simulink model "Copter_Plane_V10_sim"  (R2021a)
settings: Solver=ode1  StartTime=0.0  StopTime=10  FixedStep=dt  RelTol=1e-3
undefined symbols (not defined in the file or in its folder): AC_Attitude, AC_PosControl, accel_target, AP_Motors, curr_pos, Curr_sate, curr_vel, Euler, GRAVITY_MSS, gyro, HD, J, m_kg, Newton, pid_vel_xy_input, pos_target, position, Raphson, rho, SINS, SRV_Channel, Vehicle, vel_target, velocity
libraries: sharedutil x4, shared6dofsys x2, simulink x2, sharedtransform x2, aerolibasang x1
(part 2 of 2)

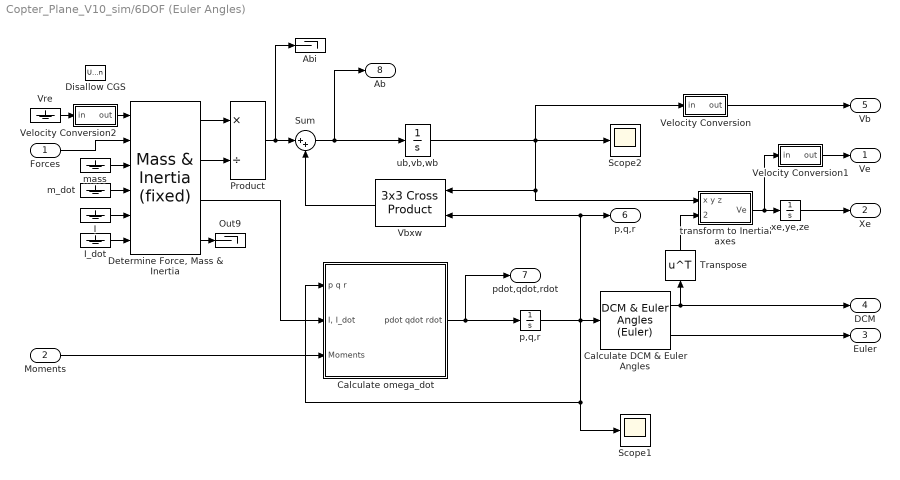
== system Copter_Plane_V10_sim/6DOF (Euler Angles) ==
  Forces : Inport  Unit=N  PortDimensions=3
  Moments : Inport  Port=2  Unit=N*m  PortDimensions=3
  Abi : Terminator
  Calculate DCM & Euler Angles : shared6dofsys/DCM & Euler Angles (Euler)  aMode=aMode
      settings: SourceProductBaseCode=AE,PW,DR,MT,UV,VE
  Calculate omega_dot : Subsystem  AncestorBlock=shared6dofsys/Calculate omega_dot  mask{aMode=aMode}
      mask init:
      | if aerosharedtest(gcb)
      |     aerosharedicon('shared');
      | else
      |     sharedautoicon('shared');
      | end
  "Determine Force, Mass & Inertia" : shared6dofsys/Mass & Inertia (fixed)  aMode=aMode
      settings: SourceProductBaseCode=AE,PW,DR,MT,UV,VE
  Disallow CGS : UnitConfiguration  UnitSystemsStr=English,SI,SI (extended)  AllowAllUnitSystems=off
  I : Ground
  I_dot : Ground
  Out9 : Terminator
  Product : Product  Inputs=*/  SaturateOnIntegerOverflow=on  OutDataTypeStr=Inherit: Same as first input
  Scope1 : Scope
  Scope2 : Scope
  Sum : Sum  Inputs=|++  SaturateOnIntegerOverflow=on
  Transpose : Math  Operator=transpose  SignedPower=on  SaturateOnIntegerOverflow=on
  Vbxw : sharedutil/3x3 Cross Product  aMode=aMode
      settings: SourceProductBaseCode=AE,PW,DR,MT,UV,VE
  Velocity Conversion : Subsystem
  Velocity Conversion1 : Subsystem
  Velocity Conversion2 : Subsystem
  Vre : Ground
  m_dot : Ground
  mass : Ground
  "p,q,r " : Integrator  InitialCondition=pm_0  ContinuousStateAttributes=pm_statename
  "transform to Inertial axes " : Subsystem  mask(Vector Transformation){}
      mask Display: disp('L_EB')
  ub,vb,wb : Integrator  InitialCondition=Vm_0  ContinuousStateAttributes=Vm_statename
  xe,ye,ze : Integrator  InitialCondition=xme_0  ContinuousStateAttributes=xme_statename
  Ve : Outport  Unit=m/s  VectorParamsAs1DForOutWhenUnconnected=off
  Xe : Outport  Port=2  Unit=m  VectorParamsAs1DForOutWhenUnconnected=off
  Euler : Outport  Port=3  Unit=rad  VectorParamsAs1DForOutWhenUnconnected=off
  DCM : Outport  Port=4  Unit=1  VectorParamsAs1DForOutWhenUnconnected=off
  Vb : Outport  Port=5  Unit=m/s  VectorParamsAs1DForOutWhenUnconnected=off
  p,q,r : Outport  Port=6  Unit=rad/s  VectorParamsAs1DForOutWhenUnconnected=off
  pdot,qdot,rdot : Outport  Port=7  Unit=rad/s^2  VectorParamsAs1DForOutWhenUnconnected=off
  Ab : Outport  Port=8  Unit=m/s^2  VectorParamsAs1DForOutWhenUnconnected=off
  wires:
  Velocity Conversion1/1(out) -> Ve/1
  Sum/1 -> Ab/1, ub,vb,wb/1
  ub,vb,wb/1 -> "transform to Inertial axes "/1(x y z), Vbxw/1, Scope2/1, Velocity Conversion/1(in)
  Velocity Conversion/1(out) -> Vb/1
  Velocity Conversion2/1(out) -> "Determine Force, Mass & Inertia"/1
  Vre/1 -> Velocity Conversion2/1(in)
  "Determine Force, Mass & Inertia"/1 -> Product/1
  I_dot/1 -> "Determine Force, Mass & Inertia"/6
  I/1 -> "Determine Force, Mass & Inertia"/5
  Calculate omega_dot/1(pdot qdot rdot) -> "p,q,r "/1, pdot,qdot,rdot/1
  "Determine Force, Mass & Inertia"/4 -> Out9/1
  m_dot/1 -> "Determine Force, Mass & Inertia"/4
  "Determine Force, Mass & Inertia"/2 -> Product/2
  mass/1 -> "Determine Force, Mass & Inertia"/3
  Transpose/1 -> "transform to Inertial axes "/2(transform coefficients)
  Calculate DCM & Euler Angles/1 -> Transpose/1, DCM/1
  Product/1 -> Sum/1, Abi/1
  Forces/1 -> "Determine Force, Mass & Inertia"/2
  Moments/1 -> Calculate omega_dot/3(Moments)
  "p,q,r "/1 -> Calculate DCM & Euler Angles/1, Scope1/1, Calculate omega_dot/1(p q r), p,q,r/1, Vbxw/2
  "transform to Inertial axes "/1(Ve) -> xe,ye,ze/1, Velocity Conversion1/1(in)
  xe,ye,ze/1 -> Xe/1
  Vbxw/1 -> Sum/2
  Calculate DCM & Euler Angles/2 -> Euler/1
  "Determine Force, Mass & Inertia"/3 -> Calculate omega_dot/2("I, I_dot")

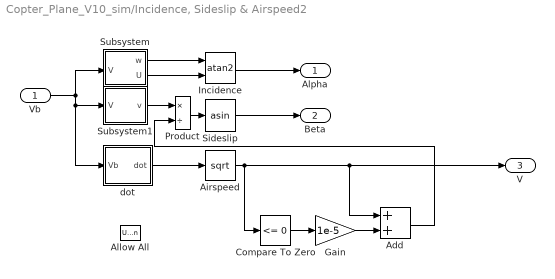
== system Copter_Plane_V10_sim/Incidence, Sideslip & Airspeed2 ==
  Vb : Inport
  Add : Sum
  Airspeed : Sqrt  AlgorithmType=Newton-Raphson  SaturateOnIntegerOverflow=on
  Allow All : UnitConfiguration  UnitSystemsStr=English,SI,SI (extended)  AllowAllUnitSystems=off
  Compare To Zero : simulink/Logic and Bit Operations/Compare To Zero  relop=<=  OutDataTypeStr=boolean
  Gain : Gain  Gain=1e-5
  Incidence : Trigonometry  Operator=atan2
  Product : Product  Inputs=*/  SaturateOnIntegerOverflow=on  OutDataTypeStr=Inherit: Same as first input
  Sideslip : Trigonometry  Operator=asin
  Subsystem : Subsystem
  Subsystem1 : Subsystem
  dot : Subsystem
  Alpha : Outport  Unit=rad  InitialOutput=0  VectorParamsAs1DForOutWhenUnconnected=off
  Beta : Outport  Port=2  Unit=rad  InitialOutput=0  VectorParamsAs1DForOutWhenUnconnected=off
  V : Outport  Port=3  InitialOutput=0  VectorParamsAs1DForOutWhenUnconnected=off
  wires:
  Product/1 -> Sideslip/1
  Subsystem/1(w) -> Incidence/1
  Subsystem/2(U) -> Incidence/2
  dot/1(dot) -> Airspeed/1
  Airspeed/1 -> Compare To Zero/1, Add/1, V/1
  Incidence/1 -> Alpha/1
  Vb/1 -> Subsystem/1(V), Subsystem1/1(V), dot/1(Vb)
  Sideslip/1 -> Beta/1
  Subsystem1/1(v) -> Product/1
  Compare To Zero/1 -> Gain/1
  Gain/1 -> Add/2
  Add/1 -> Product/2

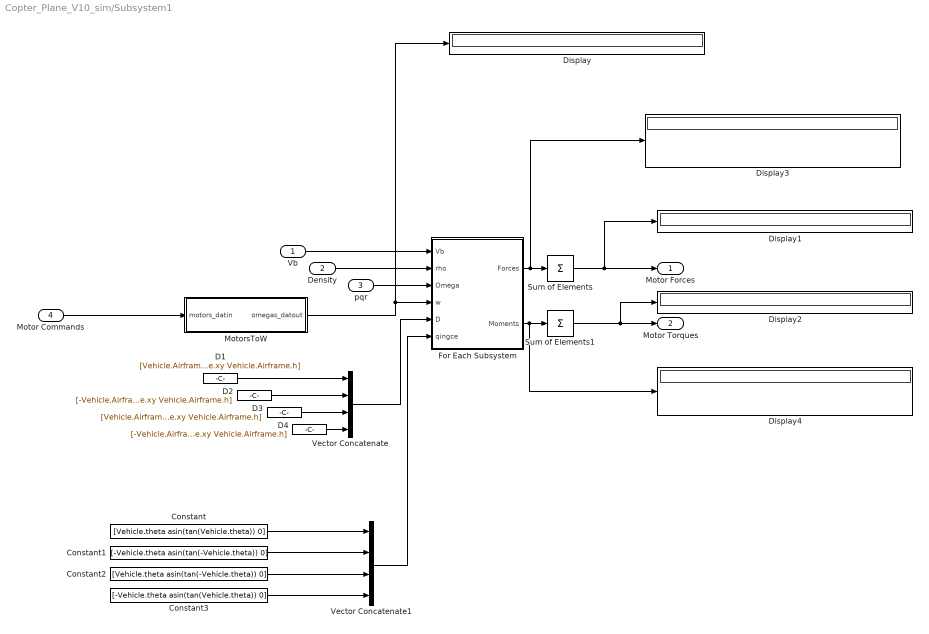
== system Copter_Plane_V10_sim/Subsystem1 ==
  Vb : Inport
  Density : Inport  Port=2
  pqr : Inport  Port=3
  Motor Commands : Inport  Port=4
  Constant : Constant  Value=[Vehicle.theta asin(tan(Vehicle.theta)) 0]
  Constant1 : Constant  Value=[-Vehicle.theta asin(tan(-Vehicle.theta)) 0]
  Constant2 : Constant  Value=[Vehicle.theta asin(tan(-Vehicle.theta)) 0]
  Constant3 : Constant  Value=[-Vehicle.theta asin(tan(Vehicle.theta)) 0]
  D1 : Constant  Value=[Vehicle.Airframe.xy +Vehicle.Airframe.xy Vehicle.Airframe.h]
  D2 : Constant  Value=[-Vehicle.Airframe.xy -Vehicle.Airframe.xy Vehicle.Airframe.h]
  D3 : Constant  Value=[Vehicle.Airframe.xy -Vehicle.Airframe.xy Vehicle.Airframe.h]
  D4 : Constant  Value=[-Vehicle.Airframe.xy Vehicle.Airframe.xy Vehicle.Airframe.h]
  Display{,1..4} (5 alike) : Display
  For Each Subsystem : Subsystem  TreatAsAtomicUnit=on
  MotorsToW : Subsystem
  Sum of Elements : Sum  Inputs=+  CollapseMode=Specified dimension  CollapseDim=2
  Sum of Elements1 : Sum  Inputs=+  CollapseMode=Specified dimension  CollapseDim=2
  Vector Concatenate : Concatenate  NumInputs=4  Mode=Multidimensional array  ConcatenateDimension=2
  Vector Concatenate1 : Concatenate  NumInputs=4  Mode=Multidimensional array  ConcatenateDimension=2
  Motor Forces : Outport  Unit=N  VectorParamsAs1DForOutWhenUnconnected=off
  Motor Torques : Outport  Port=2  Unit=N*m  VectorParamsAs1DForOutWhenUnconnected=off
  wires:
  Vector Concatenate/1 -> For Each Subsystem/5(D)
  Density/1 -> For Each Subsystem/2(rho)
  D4/1 -> Vector Concatenate/4
  Vb/1 -> For Each Subsystem/1(Vb)
  Sum of Elements1/1 -> Display2/1, Motor Torques/1
  D3/1 -> Vector Concatenate/3
  Sum of Elements/1 -> Display1/1, Motor Forces/1
  pqr/1 -> For Each Subsystem/3(Omega)
  D1/1 -> Vector Concatenate/1
  For Each Subsystem/2(Moments) -> Display4/1, Sum of Elements1/1
  For Each Subsystem/1(Forces) -> Display3/1, Sum of Elements/1
  D2/1 -> Vector Concatenate/2
  MotorsToW/1(omegas_datout) -> Display/1, For Each Subsystem/4(w)
  Motor Commands/1 -> MotorsToW/1(motors_datin)
  Vector Concatenate1/1 -> For Each Subsystem/6(qingce)
  Constant/1 -> Vector Concatenate1/1
  Constant1/1 -> Vector Concatenate1/2
  Constant2/1 -> Vector Concatenate1/3
  Constant3/1 -> Vector Concatenate1/4

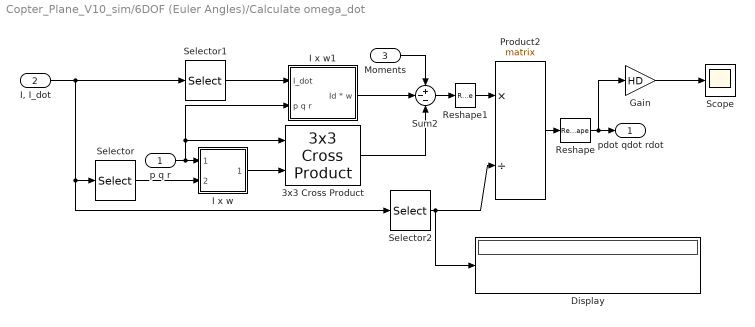
== system Copter_Plane_V10_sim/6DOF (Euler Angles)/Calculate omega_dot ==
  p q r : Inport
  "I, I_dot" : Inport  Port=2
  Moments : Inport  Port=3
  3x3 Cross Product : sharedutil/3x3 Cross Product  aMode=aMode
      settings: SourceProductBaseCode=AE,PW,DR,MT,UV,VE
  Display : Display
  Gain : Gain  Gain=HD
  I x w : Subsystem
  I x w1 : Subsystem
  Product2 : Product  Inputs=*/  Multiplication=Matrix(*)  SaturateOnIntegerOverflow=on  OutDataTypeStr=Inherit: Same as first input
  Reshape : Reshape
  Reshape1 : Reshape  OutputDimensionality=Row vector (2-D)
  Scope : Scope
  Selector : Selector  NumberOfDimensions=2  InputPortWidth=2  IndexOptions=Index vector (dialog),Select all  Indices=1:3,-1  OutputSizes=1
  Selector1 : Selector  NumberOfDimensions=2  InputPortWidth=2  IndexOptions=Index vector (dialog),Select all  Indices=4:6,-1  OutputSizes=1
  Selector2 : Selector  NumberOfDimensions=2  InputPortWidth=2  IndexOptions=Index vector (dialog),Select all  Indices=1:3,-1  OutputSizes=1
  Sum2 : Sum  Inputs=+--  SaturateOnIntegerOverflow=on
  pdot qdot rdot : Outport  VectorParamsAs1DForOutWhenUnconnected=off
  wires:
  Reshape1/1 -> Product2/1
  I x w/1(I * w) -> 3x3 Cross Product/2
  3x3 Cross Product/1 -> Sum2/3
  Selector1/1 -> I x w1/1(I_dot)
  I x w1/1(Id * w) -> Sum2/2
  Moments/1 -> Sum2/1
  Sum2/1 -> Reshape1/1
  Product2/1 -> Reshape/1
  p q r/1 -> I x w1/2(p q r), 3x3 Cross Product/1, I x w/1(p q r)
  "I, I_dot"/1 -> Selector1/1, Selector2/1, Selector/1
  Selector/1 -> I x w/2(Inertia)
  Reshape/1 -> Gain/1, pdot qdot rdot/1
  Selector2/1 -> Display/1, Product2/2
  Gain/1 -> Scope/1

== system Copter_Plane_V10_sim/6DOF (Euler Angles)/Velocity Conversion ==
  in : Inport  Unit=m/s
  Unit Conversion : UnitConversion
  out : Outport  VectorParamsAs1DForOutWhenUnconnected=off
  wires:
  Unit Conversion/1 -> out/1
  in/1 -> Unit Conversion/1

== system Copter_Plane_V10_sim/6DOF (Euler Angles)/Velocity Conversion1 ==
  in : Inport  Unit=m/s
  Unit Conversion : UnitConversion
  out : Outport  VectorParamsAs1DForOutWhenUnconnected=off
  wires:
  Unit Conversion/1 -> out/1
  in/1 -> Unit Conversion/1

== system Copter_Plane_V10_sim/6DOF (Euler Angles)/Velocity Conversion2 ==
  in : Inport  Unit=m/s
  Unit Conversion : UnitConversion
  out : Outport  Unit=m/s  VectorParamsAs1DForOutWhenUnconnected=off
  wires:
  Unit Conversion/1 -> out/1
  in/1 -> Unit Conversion/1

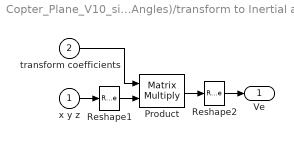
== system Copter_Plane_V10_sim/6DOF (Euler Angles)/transform to Inertial axes  ==
  x y z : Inport
  transform coefficients : Inport  Port=2
  Product : Product  Multiplication=Matrix(*)  InputSameDT=on  SaturateOnIntegerOverflow=on  OutDataTypeStr=Inherit: Same as first input
  Reshape1 : Reshape  OutputDimensionality=Column vector (2-D)
  Reshape2 : Reshape
  Ve : Outport  VectorParamsAs1DForOutWhenUnconnected=off
  wires:
  Reshape2/1 -> Ve/1
  Reshape1/1 -> Product/2
  x y z/1 -> Reshape1/1
  transform coefficients/1 -> Product/1
  Product/1 -> Reshape2/1

== system Copter_Plane_V10_sim/Incidence, Sideslip & Airspeed2/Subsystem ==
  V : Inport
  Demux1 : Demux  Outputs=3
      settings: DisplayOption=none
  Terminator : Terminator
  w : Outport  VectorParamsAs1DForOutWhenUnconnected=off
  U : Outport  Port=2  VectorParamsAs1DForOutWhenUnconnected=off
  wires:
  Demux1/3 -> w/1
  Demux1/2 -> Terminator/1
  V/1 -> Demux1/1
  Demux1/1 -> U/1

== system Copter_Plane_V10_sim/Incidence, Sideslip & Airspeed2/Subsystem1 ==
  V : Inport
  Demux1 : Demux  Outputs=3
      settings: DisplayOption=none
  Terminator : Terminator
  Terminator1 : Terminator
  v : Outport  VectorParamsAs1DForOutWhenUnconnected=off
  wires:
  Demux1/1 -> Terminator/1
  Demux1/3 -> Terminator1/1
  V/1 -> Demux1/1
  Demux1/2 -> v/1

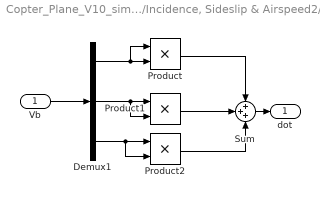
== system Copter_Plane_V10_sim/Incidence, Sideslip & Airspeed2/dot ==
  Vb : Inport
  Demux1 : Demux  Outputs=3
  Product : Product  RndMeth=Zero
  Product1 : Product  RndMeth=Zero
  Product2 : Product  RndMeth=Zero
  Sum : Sum  Inputs=+++
  dot : Outport  VectorParamsAs1DForOutWhenUnconnected=off
  wires:
  Product2/1 -> Sum/3
  Demux1/3 -> Product2/2, Product2/1
  Product/1 -> Sum/1
  Product1/1 -> Sum/2
  Sum/1 -> dot/1
  Vb/1 -> Demux1/1
  Demux1/1 -> Product/2, Product/1
  Demux1/2 -> Product1/1, Product1/2

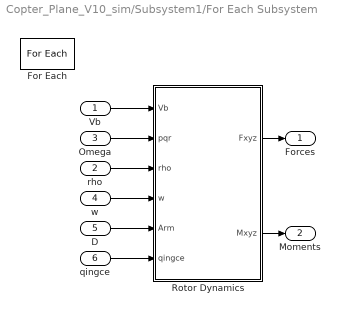
== system Copter_Plane_V10_sim/Subsystem1/For Each Subsystem ==
  Vb : Inport  PortDimensions=3
  rho : Inport  Port=2  PortDimensions=1
  Omega : Inport  Port=3
  w : Inport  Port=4  Partition=on  PartitionDimension=2  PartitionWidth=1  PartitionOffset=0
  D : Inport  Port=5  Partition=on  PartitionDimension=2  PartitionWidth=1  PartitionOffset=0
  qingce : Inport  Port=6  Partition=on  PartitionDimension=2  PartitionWidth=1  PartitionOffset=0
  For Each : ForEach  DisableCoverage=on
  Rotor Dynamics : Subsystem  AncestorBlock=dynamicsLibrary/Rotor Dynamics  TreatAsAtomicUnit=on
      mask init:
      | aeroicon('aeroblk');
      settings: RTWFcnNameOpts=Use subsystem name  RTWFileNameOpts=Use function name
  Forces : Outport  ConcatenationDimension=2  VectorParamsAs1DForOutWhenUnconnected=off
  Moments : Outport  Port=2  ConcatenationDimension=2  VectorParamsAs1DForOutWhenUnconnected=off
  wires:
  Rotor Dynamics/1(Fxyz) -> Forces/1
  Rotor Dynamics/2(Mxyz) -> Moments/1
  Vb/1 -> Rotor Dynamics/1(Vb)
  Omega/1 -> Rotor Dynamics/2(pqr)
  rho/1 -> Rotor Dynamics/3(rho)
  D/1 -> Rotor Dynamics/5(Arm)
  w/1 -> Rotor Dynamics/4(w)
  qingce/1 -> Rotor Dynamics/6(qingce)

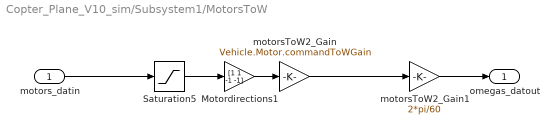
== system Copter_Plane_V10_sim/Subsystem1/MotorsToW ==
  motors_datin : Inport
  Motordirections1 : Gain  Gain=[1 1 -1 -1]  ParamDataTypeStr=single  OutDataTypeStr=Inherit: Inherit via back propagation  SaturateOnIntegerOverflow=on
  Saturation5 : Saturate  UpperLimit=1  LowerLimit=realmin  OutDataTypeStr=Inherit: Inherit via back propagation
  motorsToW2_Gain : Gain  Gain=Vehicle.Motor.commandToWGain  ParamDataTypeStr=single  OutDataTypeStr=Inherit: Inherit via back propagation  SaturateOnIntegerOverflow=on
  motorsToW2_Gain1 : Gain  Gain=2*pi/60  ParamDataTypeStr=single  OutDataTypeStr=Inherit: Inherit via back propagation  SaturateOnIntegerOverflow=on
  omegas_datout : Outport  VectorParamsAs1DForOutWhenUnconnected=off
  wires:
  Saturation5/1 -> Motordirections1/1
  Motordirections1/1 -> motorsToW2_Gain/1
  motors_datin/1 -> Saturation5/1
  motorsToW2_Gain/1 -> motorsToW2_Gain1/1
  motorsToW2_Gain1/1 -> omegas_datout/1

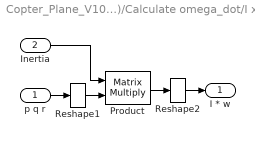
== system Copter_Plane_V10_sim/6DOF (Euler Angles)/Calculate omega_dot/I x w ==
  p q r : Inport
  Inertia : Inport  Port=2
  Product : Product  Multiplication=Matrix(*)  InputSameDT=on  SaturateOnIntegerOverflow=on  OutDataTypeStr=Inherit: Same as first input
  Reshape1 : Reshape  OutputDimensionality=Column vector (2-D)
  Reshape2 : Reshape
  I * w : Outport  VectorParamsAs1DForOutWhenUnconnected=off
  wires:
  Reshape2/1 -> I * w/1
  Reshape1/1 -> Product/2
  p q r/1 -> Reshape1/1
  Inertia/1 -> Product/1
  Product/1 -> Reshape2/1

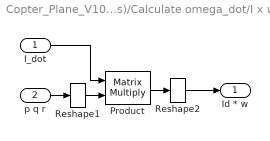
== system Copter_Plane_V10_sim/6DOF (Euler Angles)/Calculate omega_dot/I x w1 ==
  I_dot : Inport
  p q r : Inport  Port=2
  Product : Product  Multiplication=Matrix(*)  InputSameDT=on  SaturateOnIntegerOverflow=on  OutDataTypeStr=Inherit: Same as first input
  Reshape1 : Reshape  OutputDimensionality=Column vector (2-D)
  Reshape2 : Reshape
  Id * w : Outport  VectorParamsAs1DForOutWhenUnconnected=off
  wires:
  Reshape2/1 -> Id * w/1
  Reshape1/1 -> Product/2
  Product/1 -> Reshape2/1
  I_dot/1 -> Product/1
  p q r/1 -> Reshape1/1

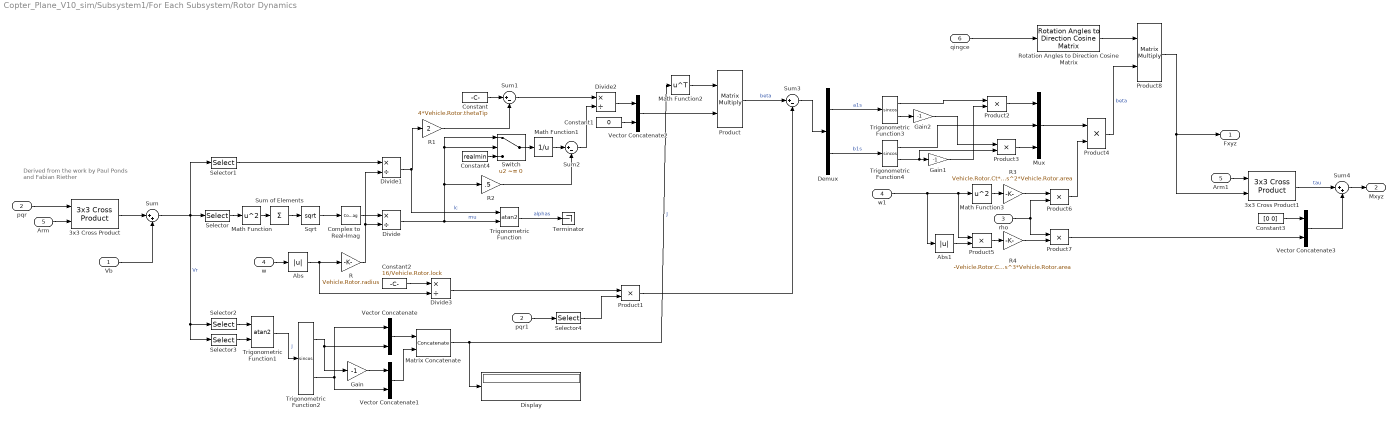
== system Copter_Plane_V10_sim/Subsystem1/For Each Subsystem/Rotor Dynamics ==
  note: Derived from the work by Paul Ponds
      | and Fabian Riether
  Vb : Inport  PortDimensions=3
  pqr : Inport  Port=2  PortDimensions=3
  rho : Inport  Port=3  PortDimensions=1
  w : Inport  Port=4  PortDimensions=[1 1]
  Arm : Inport  Port=5  PortDimensions=[3 1]
  qingce : Inport  Port=6  PortDimensions=[3 1]
  3x3 Cross Product : sharedutil/3x3 Cross Product  aMode=aMode
      settings: SourceProductBaseCode=AE,PW,DR,MT,UV,VE
  3x3 Cross Product1 : sharedutil/3x3 Cross Product  aMode=aMode
      settings: SourceProductBaseCode=AE,PW,DR,MT,UV,VE
  Abs : Abs
  Abs1 : Abs
  Arm1 : InportShadow  Port=5  PortDimensions=[3 1]
  Complex to Real-Imag : ComplexToRealImag  Output=Real
  Constant : Constant  Value=4*Vehicle.Rotor.thetaTip
  Constant1 : Constant  Value=0
  Constant2 : Constant  Value=16/Vehicle.Rotor.lock
  Constant3 : Constant  Value=[0 0]
  Constant4 : Constant  Value=realmin
  Demux : Demux  Outputs=2
  Display : Display
  Divide{,1..3} (4 alike) : Product  Inputs=*/
  Gain : Gain  Gain=-1
  Gain1 : Gain  Gain=-1
  Gain2 : Gain  Gain=-1
  Math Function : Math  Operator=square  SignedPower=on  SaturateOnIntegerOverflow=on
  Math Function1 : Math  Operator=reciprocal  SignedPower=on  SaturateOnIntegerOverflow=on
  Math Function2 : Math  Operator=transpose  SignedPower=on  SaturateOnIntegerOverflow=on
  Math Function3 : Math  Operator=square  SignedPower=on  SaturateOnIntegerOverflow=on
  Matrix Concatenate : Concatenate  Mode=Multidimensional array  ConcatenateDimension=2
  Mux : Mux  Inputs=3
  Product : Product  Multiplication=Matrix(*)
  Product{1..7} (7 alike) : Product
  Product8 : Product  Multiplication=Matrix(*)
  R : Gain  Gain=Vehicle.Rotor.radius
  R1 : Gain  Gain=2
  R2 : Gain  Gain=.5
  R3 : Gain  Gain=Vehicle.Rotor.Ct*Vehicle.Rotor.radius^2*Vehicle.Rotor.area
  R4 : Gain  Gain=-Vehicle.Rotor.Cq*Vehicle.Rotor.radius^3*Vehicle.Rotor.area
  Rotation Angles to Direction Cosine Matrix : sharedtransform/Rotation Angles to Direction Cosine Matrix  rotationOrder=YXZ  aMode=aMode
      settings: SourceProductBaseCode=AE,PW,DR,MT,UV,VE
  Selector : Selector  InputPortWidth=3  IndexOptions=Index vector (dialog)  Indices=[1 2]  OutputSizes=1
  Selector1 : Selector  InputPortWidth=3  IndexOptions=Index vector (dialog)  Indices=[3]  OutputSizes=1
  Selector2 : Selector  InputPortWidth=3  IndexOptions=Index vector (dialog)  Indices=[2]  OutputSizes=1
  Selector3 : Selector  InputPortWidth=3  IndexOptions=Index vector (dialog)  Indices=[1]  OutputSizes=1
  Selector4 : Selector  InputPortWidth=3  IndexOptions=Index vector (dialog)  Indices=[2 1]  OutputSizes=1
  Sqrt : Sqrt  OutputSignalType=complex  SaturateOnIntegerOverflow=on
  Sum : Sum  Inputs=|++
  Sum of Elements : Sum  Inputs=+
  Sum1 : Sum  Inputs=|+-
  Sum2 : Sum  Inputs=|+-
  Sum3 : Sum  Inputs=|+-
  Sum4 : Sum  Inputs=|++
  Switch : Switch  Criteria=u2 ~= 0
  Terminator : Terminator
  Trigonometric Function : Trigonometry  Operator=atan2
  Trigonometric Function1 : Trigonometry  Operator=atan2
  Trigonometric Function2 : Trigonometry  Operator=sincos
  Trigonometric Function3 : Trigonometry  Operator=sincos
  Trigonometric Function4 : Trigonometry  Operator=sincos
  Vector Concatenate{,1..3} (4 alike) : Concatenate
  pqr1 : InportShadow  Port=2  PortDimensions=3
  w1 : InportShadow  Port=4  PortDimensions=[1 1]
  Fxyz : Outport  PortDimensions=[3 1]  VectorParamsAs1DForOutWhenUnconnected=off
  Mxyz : Outport  Port=2  PortDimensions=[3 1]  VectorParamsAs1DForOutWhenUnconnected=off
  wires:
  Complex to Real-Imag/1 -> Divide/1
  Sqrt/1 -> Complex to Real-Imag/1
  Constant4/1 -> Switch/3
  Switch/1 -> Math Function1/1
  Product1/1 -> Sum3/2
  rho/1 -> Product7/1, Product6/2
  Product7/1 -> Vector Concatenate3/2
  Product6/1 -> Product4/2
  Sum4/1 -> Mxyz/1
  3x3 Cross Product1/1 -> Sum4/1  "tau"
  Arm1/1 -> 3x3 Cross Product1/1
  Vector Concatenate3/1 -> Sum4/2
  Constant3/1 -> Vector Concatenate3/1
  R4/1 -> Product7/2
  Product5/1 -> R4/1
  Abs1/1 -> Product5/2
  R3/1 -> Product6/1
  Mux/1 -> Product4/1
  Gain2/1 -> Product3/1
  Product3/1 -> Mux/3
  Trigonometric Function3/2 -> Gain2/1
  Trigonometric Function4/1 -> Mux/2
  Product2/1 -> Mux/1
  Trigonometric Function3/1 -> Product2/1
  Gain1/1 -> Product2/2
  Trigonometric Function4/2 -> Gain1/1, Product3/2
  Demux/2 -> Trigonometric Function4/1  "b1s"
  Demux/1 -> Trigonometric Function3/1  "a1s"
  Sum3/1 -> Demux/1
  Math Function3/1 -> R3/1
  w1/1 -> Math Function3/1, Product5/1, Abs1/1
  Divide3/1 -> Product1/1
  Abs/1 -> R/1, Divide3/2
  Selector4/1 -> Product1/2
  pqr1/1 -> Selector4/1
  Constant2/1 -> Divide3/1
  Product/1 -> Sum3/1  "beta"
  Math Function2/1 -> Product/1
  Vector Concatenate2/1 -> Product/2
  Constant1/1 -> Vector Concatenate2/2
  Divide2/1 -> Vector Concatenate2/1
  Sum2/1 -> Divide2/2
  R2/1 -> Sum2/2
  Math Function1/1 -> Sum2/1
  Sum1/1 -> Divide2/1
  R1/1 -> Sum1/2
  Constant/1 -> Sum1/1
  Matrix Concatenate/1 -> Display/1, Math Function2/1  "J"
  Vector Concatenate1/1 -> Matrix Concatenate/2
  Vector Concatenate/1 -> Matrix Concatenate/1
  Trigonometric Function2/1 -> Gain/1, Vector Concatenate/2
  Gain/1 -> Vector Concatenate1/1
  Trigonometric Function2/2 -> Vector Concatenate/1, Vector Concatenate1/2
  Trigonometric Function1/1 -> Trigonometric Function2/1  "j"
  Selector3/1 -> Trigonometric Function1/2
  Selector2/1 -> Trigonometric Function1/1
  Trigonometric Function/1 -> Terminator/1  "alphas"
  Divide1/1 -> Trigonometric Function/1, R1/1  "lc"
  Selector1/1 -> Divide1/1
  Divide/1 -> Trigonometric Function/2, Switch/1, Switch/2, R2/1  "mu"
  R/1 -> Divide/2, Divide1/2
  w/1 -> Abs/1
  Arm/1 -> 3x3 Cross Product/2
  pqr/1 -> 3x3 Cross Product/1
  Sum of Elements/1 -> Sqrt/1
  Math Function/1 -> Sum of Elements/1
  Selector/1 -> Math Function/1
  Sum/1 -> Selector/1, Selector1/1, Selector2/1, Selector3/1  "Vr"
  Vb/1 -> Sum/2
  3x3 Cross Product/1 -> Sum/1
  qingce/1 -> Rotation Angles to Direction Cosine Matrix/1
  Rotation Angles to Direction Cosine Matrix/1 -> Product8/1
  Product4/1 -> Product8/2  "beta"
  Product8/1 -> 3x3 Cross Product1/2, Fxyz/1

== matlab function Copter_Plane_V10_sim/MATLAB Function9 ==
  data: x_cmss input; forward output; y_cmss input; right output; yaw data_store_memory
function [forward, right]= to_body(  x_cmss,   y_cmss)  
global yaw
    forward = x_cmss * cos(yaw) + y_cmss * sin(yaw);
    right = -x_cmss * sin(yaw) + y_cmss * cos(yaw);

== matlab function Copter_Plane_V10_sim/MATLAB Function15 ==
  data: u input; y output
function y = fun(u)


y= to_euler(u);

== matlab function Copter_Plane_V10_sim/MATLAB Function16 ==
  data: u input; y output
function y = fun(u)

attitude_vehicle_quat=from_rotation_matrix(u);
y= to_euler(attitude_vehicle_quat);

== matlab function Copter_Plane_V10_sim/input_euler_angle_roll_pitch_euler_rate_yaw ==
  data: GRAVITY_MSS data_store_memory; HD data_store_memory; dt data_store_memory; LOCATION_SCALING_FACTOR_INV data_store_memory; PathModeOut_sl data_store_memory; plane_mode data_store_memory; algo_remote_ct_st data_store_memory; algo_dbg_param data_store_memory; Curr_sate data_store_memory; systime data_store_memory; Test_w data_store_memory; AC_rate_pitch_pid data_store_memory; AC_rate_roll_pid data_store_memory; AC_rate_yaw_pid data_store_memory; AC_PosControl data_store_memory; AP_rate_roll data_store_memory; AP_rate_pitch data_store_memory; AP_rate_yaw data_store_memory; AP_TECS data_store_memory; AP_L1 data_store_memory; Plane data_store_memory; SRV_Channel data_store_memory; AC_Attitude data_store_memory; AP_Motors data_store_memory; Copter_Plane data_store_memory; LOCATION_SCALING_FACTOR data_store_memory; SINS data_store_memory; SlewLimiter data_store_memory
function copter_plane_run
global plane_mode

run_remote();
load_Curr_sate();
loc_run();
load_inint();
sin_step_test();
    switch plane_mode
        case ENUM_plane_mode.V1000
            run_V1000();
        case {ENUM_plane_mode.V10 ,ENUM_plane_mode.V10s ,ENUM_plane_mode.V10_1}
            run_V10();
        otherwise
            run_V10();
    end 
run_servo_pwm_adj();

end

== matlab function Copter_Plane_V10_sim/MATLAB Function17 ==
  data: x_cmss input; forward output; y_cmss input; right output; SINS data_store_memory
function [forward, right]= to_body(  x_cmss,   y_cmss)  
global SINS
yaw =SINS.yaw;
    forward = x_cmss * cos(yaw) + y_cmss * sin(yaw);
    right = -x_cmss * sin(yaw) + y_cmss * cos(yaw);

== matlab function Copter_Plane_V10_sim/MATLAB Function ==
  data: PWM input; PWM_n output
function PWM_n      = fcn(PWM)

PWM_n=(PWM-1000)/1000;

== matlab function Copter_Plane_V10_sim/MATLAB Function1 ==
  data: k_rudder input; k_aileron input; k_throttle input; k_elevator input; wx input; wy input; wz input; alpha input; beta input; V input; Aero parameter; rho input; F output; M output
function [F,M] = fcn(k_rudder,k_aileron,k_throttle,k_elevator,wx,wy,wz,alpha,beta,V, Aero,rho)
% 
k_rudder=k_rudder/4500*30;
k_aileron=k_aileron/4500*30;
k_elevator=k_elevator/4500*30;
if(V<3)
    V=0;
end
V=0;
HD=180/pi;
% [~,~,rho,~] = atom_mode(alt+2000);
q=0.5*rho*V*V;
% alpha=constrain_value(alpha,-10/HD,12/HD);
% beta=constrain_value(beta,-10/HD,12/HD);
Sbw=[cos(alpha)*cos(beta)   -cos(alpha)*sin(beta)   -sin(alpha)
    sin(beta)               cos(beta)               0
    sin(alpha)*cos(beta)    -sin(alpha)*sin(beta)   cos(alpha)];
alpha=alpha*HD;
beta =beta* HD;
CL=interp1(Aero.CL_alpha,Aero.CL,alpha,'linear',0);
CD=interp1(Aero.CD_alpha,Aero.CD,alpha,'linear',0.25);
CC_beta=interp1(Aero.CC_beta,Aero.CC,abs(beta),'linear','extrap')*sign(beta);
CC=CC_beta+Aero.CC_dr*k_rudder;
D=q*Aero.Sref*CD;
C=q*Aero.Sref*CC;
L=q*Aero.Sref*CL;
Fw=[D; C; L];
Fb=Sbw*-Fw;
Fb=-Fw;
TF=k_throttle*Aero.Tmax;
F_Plane=Fb+[TF;0;0];

%%%%%%%%%%%%%%%%%%%%%%%%%%%%%%%%%%%%%%%%%%%%%%%%%%%%%%%%
% V-立尾
% H-平尾
% F-机身
% L-机翼

Cm_V=interp1(Aero.Cm_alpha,Aero.Cm_V,alpha,'linear','extrap');
Cm_H=interp1(Aero.Cm_alpha,Aero.Cm_H,alpha,'linear','extrap');
Cm_L=interp1(Aero.Cm_alpha,Aero.Cm_L,alpha,'linear','extrap');
Cm_F=interp1(Aero.Cm_alpha,Aero.Cm_F,alpha,'linear','extrap');
Cm_H_de=interp1(Aero.Cm_elevator,Aero.Cm_H_de,k_elevator,'linear','extrap');
Cm=Cm_V+Cm_H+Cm_L+Cm_F+Cm_H_de;

Cl_beta=interp1(Aero.beta,Aero.Cl_beta,abs(beta),'linear','extrap')*sign(beta);
Cl_da=Aero.Cl_da*k_aileron;
Cl=Cl_beta+Cl_da;

Cn_beta=interp1(Aero.beta,Aero.Cn_beta,abs(beta),'linear','extrap')*sign(beta);
Cn_dr=Aero.Cn_dr*k_rudder;
Cn=Cn_beta+Cn_dr;

l=q*Aero.Sref*Aero.Lref*Cl-0.1*wx;
m=q*Aero.Sref*Aero.Lref*Cm-0.3*wy;
n=q*Aero.Sref*Aero.Lref*Cn-0.2*wz;
M_Plane=[l ;m ;n];

F=F_Plane;
M=M_Plane;


end

== matlab function Copter_Plane_V10_sim/Location_offset1 ==
  data: center_WP input; current_loc output; ofs_north input; ofs_east input; LOCATION_SCALING_FACTOR_INV data_store_memory; HD data_store_memory
function current_loc=Location_offset( center_WP,ofs_north,  ofs_east)

current_loc=Location_offset( center_WP,ofs_north,  ofs_east);

== matlab function Copter_Plane_V10_sim/MATLAB Function2 ==
  data: x_cmss input; forward output; y_cmss input; right output; yaw data_store_memory
function [forward, right]= to_body(  x_cmss,   y_cmss)  
global yaw
    forward = x_cmss * cos(yaw) + y_cmss * sin(yaw);
    right = -x_cmss * sin(yaw) + y_cmss * cos(yaw);

== matlab function Copter_Plane_V10_sim/MATLAB Function3 ==
  data: x_cmss input; forward output; y_cmss input; right output; yaw data_store_memory
function [forward, right]= to_body(  x_cmss,   y_cmss)  
global yaw
    forward = x_cmss * cos(yaw) + y_cmss * sin(yaw);
    right = -x_cmss * sin(yaw) + y_cmss * cos(yaw);

== matlab function Copter_Plane_V10_sim/MATLAB Function4 ==
  data: x_cmss input; forward output; y_cmss input; right output; yaw data_store_memory
function [forward, right]= to_body(  x_cmss,   y_cmss)  
global yaw
    forward = x_cmss * cos(yaw) + y_cmss * sin(yaw);
    right = -x_cmss * sin(yaw) + y_cmss * cos(yaw);

== matlab function Copter_Plane_V10_sim/MATLAB Function6 ==
  data: x_cmss input; forward output; y_cmss input; right output; yaw data_store_memory
function [forward, right]= to_body(  x_cmss,   y_cmss)  
global yaw
    forward = x_cmss * cos(yaw) + y_cmss * sin(yaw);
    right = -x_cmss * sin(yaw) + y_cmss * cos(yaw);

== matlab function Copter_Plane_V10_sim/get_vector_xy_from_origin_NE1 ==
  data: loc input; vec_ne output; loc_origin input; LOCATION_SCALING_FACTOR_INV data_store_memory; HD data_store_memory; LOCATION_SCALING_FACTOR data_store_memory
function vec_ne=get_vector_xy_from_origin_NE( loc,loc_origin) 

vec_ne=get_vector_xy_from_origin_NE( loc,loc_origin ) ;

== matlab function Copter_Plane_V10_sim/MATLAB Function10 ==
  data: x_cmss input; forward output; y_cmss input; right output; yaw data_store_memory
function [forward, right]= to_body(  x_cmss,   y_cmss)  
global yaw
    forward = x_cmss * cos(yaw) + y_cmss * sin(yaw);
    right = -x_cmss * sin(yaw) + y_cmss * cos(yaw);

== matlab function Copter_Plane_V10_sim/MATLAB Function5 ==
  data: x_cmss input; forward output; y_cmss input; right output; yaw data_store_memory
function [forward, right]= to_body(  x_cmss,   y_cmss)  
global yaw
    forward = x_cmss * cos(yaw) + y_cmss * sin(yaw);
    right = -x_cmss * sin(yaw) + y_cmss * cos(yaw);

== matlab function Copter_Plane_V10_sim/MATLAB Function11 ==
  data: x_cmss input; forward output; y_cmss input; right output; yaw data_store_memory
function [forward, right]= to_body(  x_cmss,   y_cmss)  
global yaw
    forward = x_cmss * cos(yaw) + y_cmss * sin(yaw);
    right = -x_cmss * sin(yaw) + y_cmss * cos(yaw);

== matlab function Copter_Plane_V10_sim/MATLAB Function13 ==
  data: x_cmss input; forward output; y_cmss input; right output; yaw data_store_memory
function [forward, right]= to_body(  x_cmss,   y_cmss)  
global yaw
    forward = x_cmss * cos(yaw) + y_cmss * sin(yaw);
    right = -x_cmss * sin(yaw) + y_cmss * cos(yaw);

== matlab function Copter_Plane_V10_sim/MATLAB Function7 ==
  data: x_cmss input; forward output; y_cmss input; right output; yaw data_store_memory
function [forward, right]= to_body(  x_cmss,   y_cmss)  
global yaw
    forward = x_cmss * cos(yaw) + y_cmss * sin(yaw);
    right = -x_cmss * sin(yaw) + y_cmss * cos(yaw);

== matlab function Copter_Plane_V10_sim/MATLAB Function8 ==
  data: x_cmss input; forward output; y_cmss input; right output; yaw data_store_memory
function [forward, right]= to_body(  x_cmss,   y_cmss)  
global yaw
    forward = x_cmss * cos(yaw) + y_cmss * sin(yaw);
    right = -x_cmss * sin(yaw) + y_cmss * cos(yaw);

== matlab function Copter_Plane_V10_sim/MATLAB Function12 ==
  data: x_cmss input; forward output; y_cmss input; right output; yaw data_store_memory
function [forward, right]= to_body(  x_cmss,   y_cmss)  
global yaw
    forward = x_cmss * cos(yaw) + y_cmss * sin(yaw);
    right = -x_cmss * sin(yaw) + y_cmss * cos(yaw);
